simulink model "DAB Converters ude vr"  (R2022a)
settings: Solver=VariableStepAuto  StartTime=0.0  StopTime=0.5  RelTol=1e-3
libraries: spsMosfetLib x16, spsSeriesRLCBranchLib x6, spsVoltageMeasurementLib x6, spsCurrentMeasurementLib x4, simulink_extras x4, spsSawtoothGeneratorLib x4, spspowerguiLib x3, spsControlledVoltageSourceLib x2, spsLinearTransformerLib x2, spsControlledCurrentSourceLib x2, slpidlib x1
settings Model: Creator=shuai  LastModifiedBy=shuai

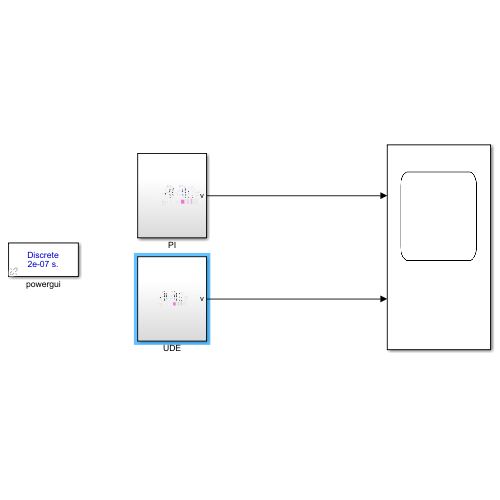
[thumbnail: Simulink's stored preview of the top-level diagram]
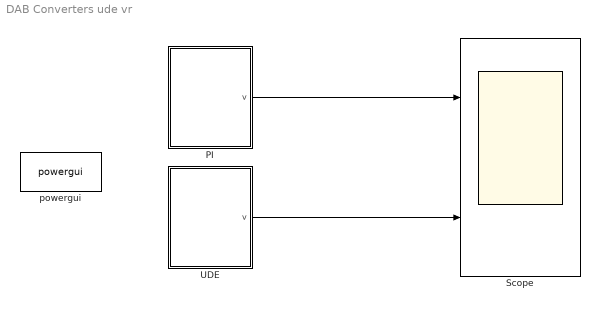
== system DAB Converters ude vr ==
  PI : Subsystem
  Scope : Scope  NumInputPorts=2
  UDE : Subsystem
  powergui : spspowerguiLib/powergui  Priority=1  SimulationMode=Discrete  SampleTime=2e-7  frequency=60  Iterations=50  frequencyindice=0  Pbase=100e6  ErrMax=1e-4  UnitsV=kV  UnitsW=MW  buscounter=0  FunctionMessages=off  echomessages=off  EnableUseOfTLC=off  CurrentSourceSwitches=off  DisableSnubberDevices=off  DisableRonSwitches=off  DisableVfSwitches=off  DisplayEquations=off  AutomaticDiscreteSolvers=off  SolverType=Tustin/Backward Euler (TBE)  Interpol=off  ExternalGateDelay=off  methode=off  Ts=100  x0status=blocks  SPID=on  SwTol=0  HookPort=off  NonlinearTolerance=1e-4  nMaxIteration=100  ContinueOnMaxIteration=off  RestoreLinks=warning  ResistiveCurrentMeasurement=off  Frange=[0:2:500]  Ylog=off  Xlog=on  ShowGrid=off  save=off  variable=ZData  structure=0  ZoomFFT=off  StartTime=0.0  cycles=1  DisplayStyle=1  fundamental=60  FreqAxis=off  MaxFrequency=1000  frequencyindicesteady=1  RmsSteady=1  display=off
  wires:
  PI/1(v) -> Scope/1
  UDE/1(v) -> Scope/2

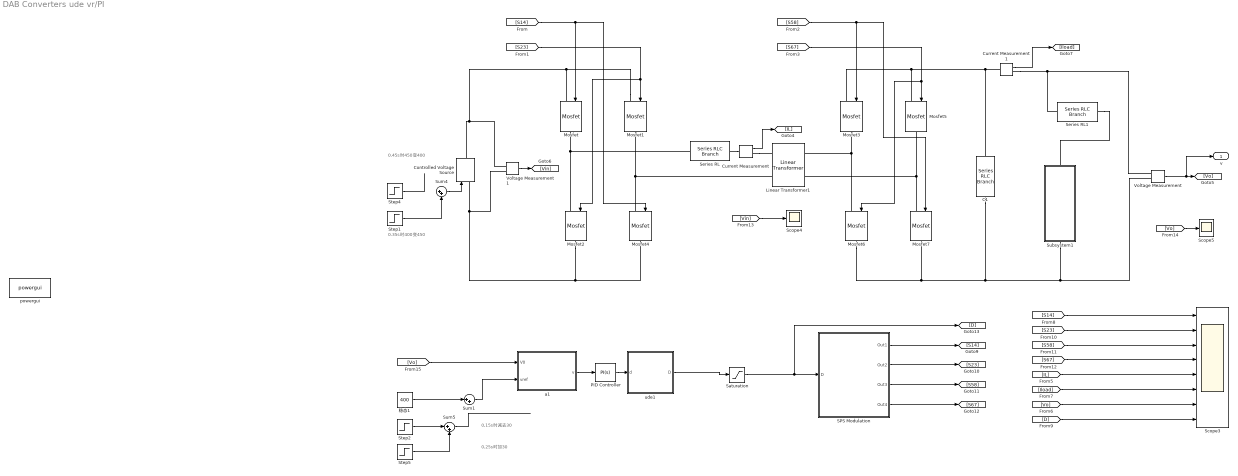
== system DAB Converters ude vr/PI ==
  note: 0.35s时400变450
  note: 0.45s时450变400
  note: 0,25s时加30
  note: 0,15s时减去30
  C1 : spsSeriesRLCBranchLib/Series RLC Branch  LConnTagsString=__new0  RConnTagsString=__new0  BranchType=C  Resistance=0.01  Inductance=1e-3  SetiL0=off  InitialCurrent=0  Capacitance=400e-6  Setx0=on  InitialVoltage=0  Measurements=None
  Controlled Voltage Source : spsControlledVoltageSourceLib/Controlled Voltage Source  Initialize=on  Source_Type=DC  Amplitude=0  Phase=0  Frequency=0  Measurements=None
  Current Measurement : spsCurrentMeasurementLib/Current Measurement  PhasorSimulation=off  OutputType=Complex  PSBequivalent=0
  Current Measurement1 : spsCurrentMeasurementLib/Current Measurement  PhasorSimulation=off  OutputType=Complex  PSBequivalent=0
  Linear Transformer1 : spsLinearTransformerLib/Linear Transformer  UNITS=SI  NominalPower=[20e5 20000 ]  winding1=[1000 0 0]  winding2=[1000 0 0]  ThreeWindings=off  winding3=[3.15e+05 39690 12.634]  RmLm=[8.5e4 8.5e4]  Measurements=None  DataType=on
  Mosfet{,1..7} (8 alike) : spsMosfetLib/Mosfet  Ron=0.001  Lon=0  Rd=0.001  Vfd=0  IC=0  Rs=1e5  Cs=inf  Measurements=off
  PID Controller : slpidlib/PID Controller  Controller=PI  Form=Parallel  TimeDomain=Continuous-time  UseExternalTs=off  SampleTime=-1  IntegratorMethod=Forward Euler  FilterMethod=Forward Euler  ControllerParametersSource=internal  P=0.000544489  I=0.116994  UseKiTs=off  D=0  N=100  UseFilter=on  TunerSelectOption=Transfer Function Based (PID Tuner App)  InitialConditionSource=internal  InitialConditionForIntegrator=0  InitialConditionForFilter=0  DifferentiatorICPrevScaledInput=0  ExternalReset=none  TrackingMode=off  Kt=1  LimitOutput=off  SatLimitsSource=internal  UpperSaturationLimit=inf  LowerSaturationLimit=-inf  LinearizeAsGain=on  AntiWindupMode=none  Kb=1  POutMin=[]  POutMax=[]  IOutMin=[]  IOutMax=[]  DOutMin=[]  DOutMax=[]  NOutMin=[]  NOutMax=[]  SumOutMin=[]  SumOutMax=[]  SaturationOutMin=[]  SaturationOutMax=[]  PParamMin=[]  PParamMax=[]  IParamMin=[]  IParamMax=[]  DParamMin=[]  DParamMax=[]  NParamMin=[]  NParamMax=[]  KbParamMin=[]  KbParamMax=[]  KtParamMin=[]  KtParamMax=[]  KbOutMin=[]  KbOutMax=[]  KtOutMin=[]  KtOutMax=[]  IntegratorOutMin=[]  IntegratorOutMax=[]  FilterOutMin=[]  FilterOutMax=[]  SumI1OutMin=[]  SumI1OutMax=[]  SumI2OutMin=[]  SumI2OutMax=[]  SumI3OutMin=[]  SumI3OutMax=[]  SumI4OutMin=[]  SumI4OutMax=[]  SumDOutMin=[]  SumDOutMax=[]  DifferentiatorOutMin=[]  DifferentiatorOutMax=[]  FilterDiffOutCoefMin=[]  FilterDiffOutCoefMax=[]  ReciprocalOutMin=[]  ReciprocalOutMax=[]  SumDenOutMin=[]  SumDenOutMax=[]  SumNumOutMin=[]  SumNumOutMax=[]  DivideOutMin=[]  DivideOutMax=[]  UdiffTsProdOutMin=[]  UdiffTsProdOutMax=[]  NTsProdOutMin=[]  NTsProdOutMax=[]  UintegralTsProdOutMin=[]  UintegralTsProdOutMax=[]  UngainTsProdOutMin=[]  UngainTsProdOutMax=[]  IntegratorContinuousStateAttributes=''  IntegratorStateMustResolveToSignalObject=off  IntegratorRTWStateStorageClass=Auto  FilterContinuousStateAttributes=''  FilterStateMustResolveToSignalObject=off  FilterRTWStateStorageClass=Auto  ParallelPVariant=InternalParameters  IdealPVariant=Disabled  IVariant=InternalParameters  DVariant=Disabled  IntegratorVariant=Continuous  SatVariant=Disabled  AWVariant=Passthrough  PCopyVariant=Disabled  TRVariant=Disabled  FdbkBlocksVariant=Forward  IdealPFdbkVariant=Disabled  SatFdbkVariant=Disabled  DerivativeFilterVariant=Disabled  NVariant=Disabled  NCopyVariant=Disabled_SignalSpec  FilterICVariant=Disabled  IntegratorICVariant=InternalICs  ExternalResetVariant=Disabled  TRSumVariant=Passthrough  SumFdbkVariant=Disabled  SumVariant=Sum_PI  TsampFilterVariant=InternalTs  TsampNgainVariant=Passthrough  TsampIntegralVariant=Passthrough  ExternalSaturationOutDataTypeStr=Inherit: Same as second input  aMode=0
  SPS Modulation : Subsystem
  Saturation : Saturate  UpperLimit=0.9  LowerLimit=0
  Scope3 : Scope  NumInputPorts=8
  Scope4 : Scope
  Scope5 : Scope
  Series RL : spsSeriesRLCBranchLib/Series RLC Branch  LConnTagsString=__new0  RConnTagsString=__new0  BranchType=L  Resistance=0  Inductance=50e-6  SetiL0=off  InitialCurrent=0  Capacitance=1e-6  Setx0=off  InitialVoltage=0  Measurements=None
  Series RL1 : spsSeriesRLCBranchLib/Series RLC Branch  LConnTagsString=__new0  RConnTagsString=__new0  BranchType=R  Resistance=0.0001  Inductance=50e-6  SetiL0=off  InitialCurrent=0  Capacitance=1e-6  Setx0=off  InitialVoltage=0  Measurements=None
  Step1 : Step  Time=0.3  Before=400  After=400  SampleTime=0
  Step2 : Step  Time=0.1  After=-30  SampleTime=0
  Step4 : Step  Time=0.4  After=-50  SampleTime=0
  Step5 : Step  Time=0.2  After=50  SampleTime=0
  Subsystem1 : Subsystem
  Sum1 : Sum  Inputs=|++
  Sum4 : Sum  Inputs=|++
  Sum5 : Sum  Inputs=|++
  Voltage Measurement : spsVoltageMeasurementLib/Voltage Measurement  PhasorSimulation=off  OutputType=Complex  PSBequivalent=0
  Voltage Measurement1 : spsVoltageMeasurementLib/Voltage Measurement  PhasorSimulation=off  OutputType=Complex  PSBequivalent=0
  a1 : MATLAB Function  TreatAsAtomicUnit=on  SystemSampleTime=1/20000
  powergui : spspowerguiLib/powergui  Priority=1  SimulationMode=Discrete  SampleTime=2e-7  frequency=60  Iterations=50  frequencyindice=0  Pbase=100e6  ErrMax=1e-4  UnitsV=kV  UnitsW=MW  buscounter=0  FunctionMessages=off  echomessages=off  EnableUseOfTLC=off  CurrentSourceSwitches=off  DisableSnubberDevices=off  DisableRonSwitches=off  DisableVfSwitches=off  DisplayEquations=off  AutomaticDiscreteSolvers=off  SolverType=Tustin/Backward Euler (TBE)  Interpol=off  ExternalGateDelay=off  methode=off  Ts=100  x0status=blocks  SPID=off  SwTol=0  HookPort=off  NonlinearTolerance=1e-4  nMaxIteration=100  ContinueOnMaxIteration=off  RestoreLinks=warning  ResistiveCurrentMeasurement=off  Frange=[0:2:500]  Ylog=off  Xlog=on  ShowGrid=off  save=off  variable=ZData  structure=0  ZoomFFT=off  StartTime=0.0  cycles=1  DisplayStyle=1  fundamental=60  FreqAxis=off  MaxFrequency=1000  frequencyindicesteady=1  RmsSteady=1  display=off
  ude1 : MATLAB Function  TreatAsAtomicUnit=on  SystemSampleTime=1/20000
  稳态1 : Constant  Value=400  VectorParams1D=off
  v : Outport
  wires:
  SPS Modulation/4(Out4) -> [S67]
  [S23] -> Scope3/2
  Current Measurement1/1 -> [Iload]
  [S67] -> Mosfet6/1, Mosfet5/1
  SPS Modulation/3(Out3) -> [S58]
  [S58] -> Mosfet7/1, Mosfet3/1
  [S14] -> Scope3/1
  [Vin] -> Scope4/1
  Current Measurement/1 -> [IL]
  Sum4/1 -> Controlled Voltage Source/1
  [D] -> Scope3/8
  Step4/1 -> ?
  Voltage Measurement1/1 -> [Vin]
  [Vo] -> Scope5/1
  Saturation/1 -> [D], SPS Modulation/1(D)
  [S23] -> Mosfet2/1, Mosfet1/1
  Voltage Measurement/1 -> v/1, [Vo]
  SPS Modulation/2(Out2) -> [S23]
  [S14] -> Mosfet4/1, Mosfet/1
  SPS Modulation/1(Out1) -> [S14]
  [S67] -> Scope3/4
  [Iload] -> Scope3/6
  [S58] -> Scope3/3
  Step1/1 -> Sum4/2
  [IL] -> Scope3/5
  [Vo] -> Scope3/7
  Step2/1 -> Sum5/1
  Step5/1 -> Sum5/2
  Sum5/1 -> ?
  稳态1/1 -> Sum1/1
  [Vo] -> a1/1(V0)
  a1/1(v) -> PID Controller/1
  Sum1/1 -> a1/2(vref)
  PID Controller/1 -> ude1/1(d)
  ude1/1(D) -> Saturation/1
  connections:
  Mosfet1/LConn1 -- Voltage Measurement1/LConn1 -- Controlled Voltage Source/RConn1 -- Mosfet/LConn1
  Mosfet4/RConn1 -- Voltage Measurement1/LConn2 -- Controlled Voltage Source/LConn1 -- Mosfet2/RConn1
  Linear Transformer1/RConn2 -- Mosfet7/LConn1 -- Mosfet5/RConn1
  Current Measurement1/LConn1 -- C1/LConn1 -- Mosfet5/LConn1 -- Mosfet3/LConn1
  Current Measurement1/RConn1 -- Series RL1/LConn1 -- Voltage Measurement/LConn1
  Series RL/RConn1 -- Current Measurement/LConn1
  Mosfet2/LConn1 -- Mosfet/RConn1 -- Series RL/LConn1
  Mosfet1/RConn1 -- Mosfet4/LConn1 -- Linear Transformer1/LConn2
  Current Measurement/RConn1 -- Linear Transformer1/LConn1
  Linear Transformer1/RConn1 -- Mosfet6/LConn1 -- Mosfet3/RConn1
  C1/RConn1 -- Mosfet6/RConn1 -- Mosfet7/RConn1 -- Subsystem1/RConn1 -- Voltage Measurement/LConn2
  Series RL1/RConn1 -- Subsystem1/LConn1

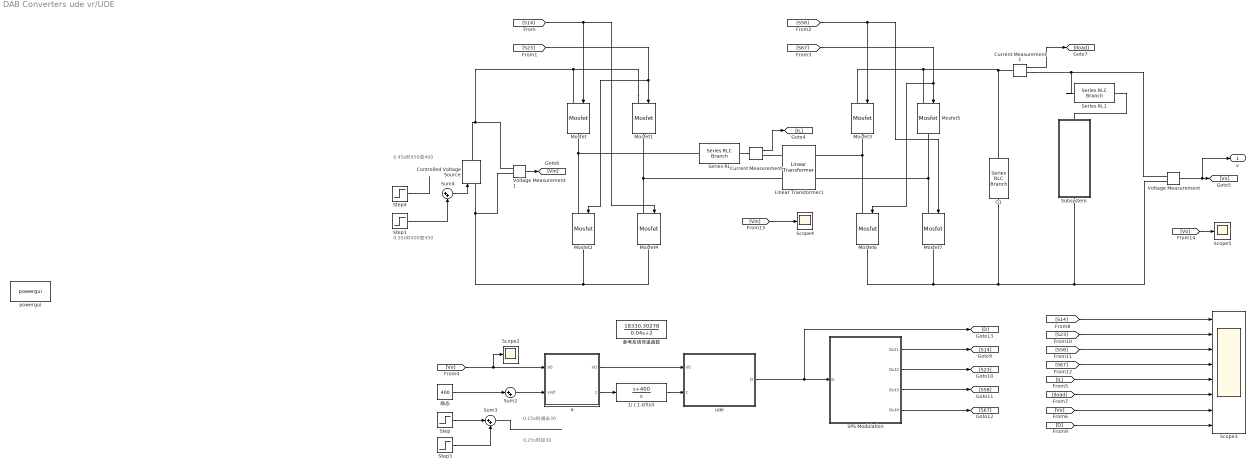
== system DAB Converters ude vr/UDE ==
  note: 0.35s时400变450
  note: 0,15s时减去30
  note: 0,25s时加30
  note: 0.45s时450变400
  1/（1-Gf(s)) : TransferFcn  Numerator=[1 400]  Denominator=[1 0]
  C1 : spsSeriesRLCBranchLib/Series RLC Branch  LConnTagsString=__new0  RConnTagsString=__new0  BranchType=C  Resistance=0.01  Inductance=1e-3  SetiL0=off  InitialCurrent=0  Capacitance=400e-6  Setx0=on  InitialVoltage=0  Measurements=None
  Controlled Voltage Source : spsControlledVoltageSourceLib/Controlled Voltage Source  Initialize=on  Source_Type=DC  Amplitude=0  Phase=0  Frequency=0  Measurements=None
  Current Measurement : spsCurrentMeasurementLib/Current Measurement  PhasorSimulation=off  OutputType=Complex  PSBequivalent=0
  Current Measurement1 : spsCurrentMeasurementLib/Current Measurement  PhasorSimulation=off  OutputType=Complex  PSBequivalent=0
  Linear Transformer1 : spsLinearTransformerLib/Linear Transformer  UNITS=SI  NominalPower=[20e5 20000 ]  winding1=[1000 0 0]  winding2=[1000 0 0]  ThreeWindings=off  winding3=[3.15e+05 39690 12.634]  RmLm=[8.5e4 8.5e4]  Measurements=None  DataType=on
  Mosfet{,1..7} (8 alike) : spsMosfetLib/Mosfet  Ron=0.001  Lon=0  Rd=0.001  Vfd=0  IC=0  Rs=1e5  Cs=inf  Measurements=off
  SPS Modulation : Subsystem
  Scope2 : Scope
  Scope3 : Scope  NumInputPorts=8
  Scope4 : Scope
  Scope5 : Scope
  Series RL : spsSeriesRLCBranchLib/Series RLC Branch  LConnTagsString=__new0  RConnTagsString=__new0  BranchType=L  Resistance=0  Inductance=50e-6  SetiL0=off  InitialCurrent=0  Capacitance=1e-6  Setx0=off  InitialVoltage=0  Measurements=None
  Series RL1 : spsSeriesRLCBranchLib/Series RLC Branch  LConnTagsString=__new0  RConnTagsString=__new0  BranchType=R  Resistance=0.0001  Inductance=50e-6  SetiL0=off  InitialCurrent=0  Capacitance=1e-6  Setx0=off  InitialVoltage=0  Measurements=None
  Step : Step  Time=0.1  After=-30  SampleTime=0
  Step1 : Step  Time=0.3  Before=400  After=400  SampleTime=0
  Step3 : Step  Time=0.2  After=50  SampleTime=0
  Step4 : Step  Time=0.4  After=-50  SampleTime=0
  Subsystem : Subsystem
  Sum2 : Sum  Inputs=|++
  Sum3 : Sum  Inputs=|++
  Sum4 : Sum  Inputs=|++
  Voltage Measurement : spsVoltageMeasurementLib/Voltage Measurement  PhasorSimulation=off  OutputType=Complex  PSBequivalent=0
  Voltage Measurement1 : spsVoltageMeasurementLib/Voltage Measurement  PhasorSimulation=off  OutputType=Complex  PSBequivalent=0
  a : MATLAB Function  TreatAsAtomicUnit=on  SystemSampleTime=1/20000
  powergui : spspowerguiLib/powergui  Priority=1  SimulationMode=Discrete  SampleTime=2e-7  frequency=60  Iterations=50  frequencyindice=0  Pbase=100e6  ErrMax=1e-4  UnitsV=kV  UnitsW=MW  buscounter=0  FunctionMessages=off  echomessages=off  EnableUseOfTLC=off  CurrentSourceSwitches=off  DisableSnubberDevices=off  DisableRonSwitches=off  DisableVfSwitches=off  DisplayEquations=off  AutomaticDiscreteSolvers=off  SolverType=Tustin/Backward Euler (TBE)  Interpol=off  ExternalGateDelay=off  methode=off  Ts=100  x0status=blocks  SPID=off  SwTol=0  HookPort=off  NonlinearTolerance=1e-4  nMaxIteration=100  ContinueOnMaxIteration=off  RestoreLinks=warning  ResistiveCurrentMeasurement=off  Frange=[0:2:500]  Ylog=off  Xlog=on  ShowGrid=off  save=off  variable=ZData  structure=0  ZoomFFT=off  StartTime=0.0  cycles=1  DisplayStyle=1  fundamental=60  FreqAxis=off  MaxFrequency=1000  frequencyindicesteady=1  RmsSteady=1  display=off
  ude : MATLAB Function  TreatAsAtomicUnit=on  SystemSampleTime=1/20000
  参考系统传递函数 : TransferFcn  Numerator=[18330.30278]  Denominator=[0.04 2]
  稳态 : Constant  Value=400  VectorParams1D=off
  v : Outport
  wires:
  SPS Modulation/4(Out4) -> [S67]
  [S23] -> Scope3/2
  Current Measurement1/1 -> [Iload]
  [S67] -> Mosfet6/1, Mosfet5/1
  SPS Modulation/3(Out3) -> [S58]
  [S58] -> Mosfet7/1, Mosfet3/1
  [S14] -> Scope3/1
  [Vin] -> Scope4/1
  Current Measurement/1 -> [IL]
  Sum4/1 -> Controlled Voltage Source/1
  [D] -> Scope3/8
  1/（1-Gf(s))/1 -> ude/2(z)
  稳态/1 -> Sum2/1
  Sum2/1 -> a/2(vref)
  Step4/1 -> ?
  Voltage Measurement1/1 -> [Vin]
  [Vo] -> Scope5/1
  ude/1(D) -> [D], SPS Modulation/1(D)
  [S23] -> Mosfet2/1, Mosfet1/1
  a/1(V0) -> ude/1(V0)
  Step/1 -> Sum3/1
  Voltage Measurement/1 -> v/1, [Vo]
  a/2(z) -> 1/（1-Gf(s))/1
  SPS Modulation/2(Out2) -> [S23]
  [S14] -> Mosfet4/1, Mosfet/1
  SPS Modulation/1(Out1) -> [S14]
  [S67] -> Scope3/4
  [Iload] -> Scope3/6
  [S58] -> Scope3/3
  Step1/1 -> Sum4/2
  [Vo] -> a/1("V0 "), Scope2/1
  Sum3/1 -> ?
  Step3/1 -> Sum3/2
  [IL] -> Scope3/5
  [Vo] -> Scope3/7
  connections:
  Mosfet1/LConn1 -- Voltage Measurement1/LConn1 -- Controlled Voltage Source/RConn1 -- Mosfet/LConn1
  Mosfet4/RConn1 -- Voltage Measurement1/LConn2 -- Controlled Voltage Source/LConn1 -- Mosfet2/RConn1
  Linear Transformer1/RConn2 -- Mosfet7/LConn1 -- Mosfet5/RConn1
  Current Measurement1/LConn1 -- C1/LConn1 -- Mosfet5/LConn1 -- Mosfet3/LConn1
  Series RL/RConn1 -- Current Measurement/LConn1
  Mosfet2/LConn1 -- Series RL/LConn1 -- Mosfet/RConn1
  Mosfet1/RConn1 -- Mosfet4/LConn1 -- Linear Transformer1/LConn2
  Current Measurement/RConn1 -- Linear Transformer1/LConn1
  Linear Transformer1/RConn1 -- Mosfet6/LConn1 -- Mosfet3/RConn1
  C1/RConn1 -- Mosfet6/RConn1 -- Mosfet7/RConn1 -- Voltage Measurement/LConn2 -- Subsystem/RConn1
  Current Measurement1/RConn1 -- Series RL1/LConn1 -- Voltage Measurement/LConn1
  Series RL1/RConn1 -- Subsystem/LConn1

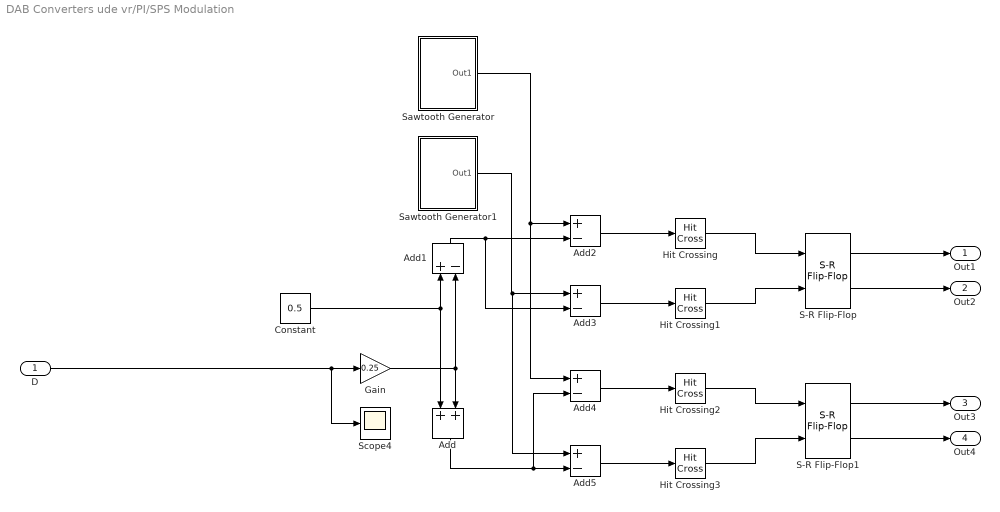
== system DAB Converters ude vr/PI/SPS Modulation ==
  D : Inport
  Add : Sum
  Add{1..5} (5 alike) : Sum  Inputs=+-
  Constant : Constant  Value=0.5
  Gain : Gain  Gain=0.25
  Hit Crossing{,1..3} (4 alike) : HitCross  HitCrossingDirection=rising
  S-R Flip-Flop : simulink_extras/Flip Flops/S-R Flip-Flop  initial_condition=0
  S-R Flip-Flop1 : simulink_extras/Flip Flops/S-R Flip-Flop  initial_condition=0
  Sawtooth Generator : Subsystem  mask{fs=20000}
      mask prompts: fs "Frequency (Hz)"
      mask help: Sawtooth Generator
  Sawtooth Generator1 : Subsystem  mask{fs=20000}
      mask prompts: fs "Frequency (Hz)"
      mask help: Sawtooth Generator
  Scope4 : Scope
  Out1 : Outport  VectorParamsAs1DForOutWhenUnconnected=off
  Out2 : Outport  Port=2  VectorParamsAs1DForOutWhenUnconnected=off
  Out3 : Outport  Port=3  VectorParamsAs1DForOutWhenUnconnected=off
  Out4 : Outport  Port=4  VectorParamsAs1DForOutWhenUnconnected=off
  wires:
  Hit Crossing1/1 -> S-R Flip-Flop/2
  Add1/1 -> Add3/2, Add2/2
  Constant/1 -> Add1/1, Add/1
  Add5/1 -> Hit Crossing3/1
  Gain/1 -> Add1/2, Add/2
  D/1 -> Gain/1, Scope4/1
  Add/1 -> Add4/2, Add5/2
  Sawtooth Generator/1(Out1) -> Add4/1, Add2/1
  Hit Crossing/1 -> S-R Flip-Flop/1
  Add2/1 -> Hit Crossing/1
  Sawtooth Generator1/1(Out1) -> Add5/1, Add3/1
  Add3/1 -> Hit Crossing1/1
  Add4/1 -> Hit Crossing2/1
  Hit Crossing2/1 -> S-R Flip-Flop1/1
  Hit Crossing3/1 -> S-R Flip-Flop1/2
  S-R Flip-Flop1/1 -> Out3/1
  S-R Flip-Flop1/2 -> Out4/1
  S-R Flip-Flop/1 -> Out1/1
  S-R Flip-Flop/2 -> Out2/1

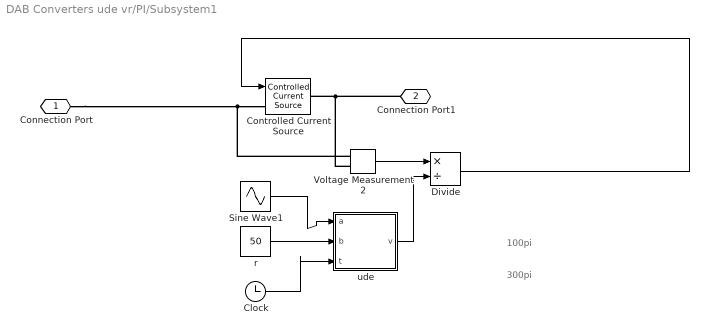
== system DAB Converters ude vr/PI/Subsystem1 ==
  note: 300pi
  note: 100pi
  Clock : Clock
  Controlled Current Source : spsControlledCurrentSourceLib/Controlled Current Source  Initialize=on  Source_Type=AC  Amplitude=0  Phase=0  Frequency=0  Measurements=None
  Divide : Product  Inputs=*/  RndMeth=Zero  SaturateOnIntegerOverflow=on
  Sine Wave1 : Sin  Amplitude=10  Bias=50  Frequency=100*pi  Samples=1e5  SampleTime=0
  Voltage Measurement2 : spsVoltageMeasurementLib/Voltage Measurement  PhasorSimulation=off  OutputType=Complex  PSBequivalent=0
  r : Constant  Value=50  VectorParams1D=off
  ude : MATLAB Function  TreatAsAtomicUnit=on  SystemSampleTime=1/20000
  Connection Port : PMIOPort  Side=Left
  Connection Port1 : PMIOPort  Port=2  Side=Right
  wires:
  Voltage Measurement2/1 -> Divide/1
  Sine Wave1/1 -> ude/1(a)
  Divide/1 -> Controlled Current Source/1
  Clock/1 -> ude/3(t)
  r/1 -> ude/2(b)
  ude/1(v) -> Divide/2
  connections:
  Voltage Measurement2/LConn2 -- Connection Port1/RConn1 -- Controlled Current Source/RConn1
  Voltage Measurement2/LConn1 -- Connection Port/RConn1 -- Controlled Current Source/LConn1

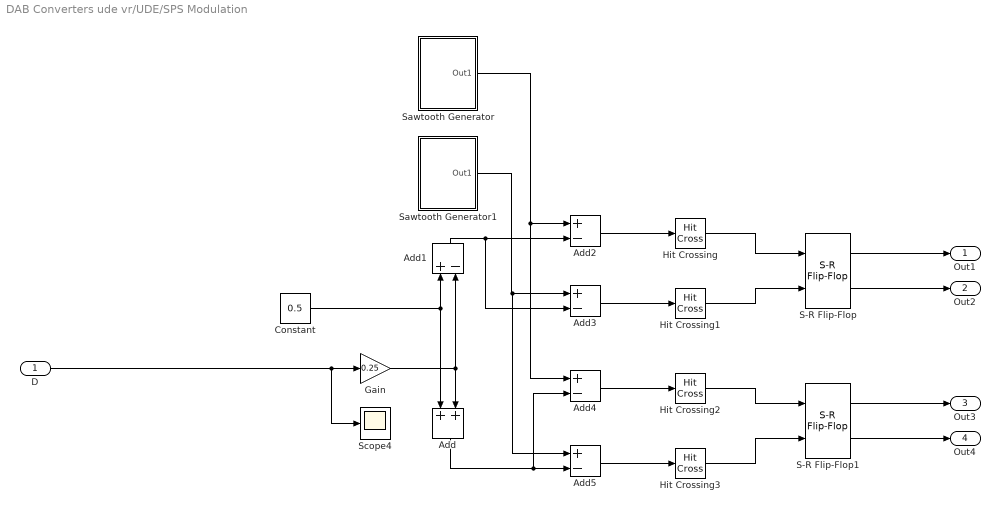
== system DAB Converters ude vr/UDE/SPS Modulation ==
  D : Inport
  Add : Sum
  Add{1..5} (5 alike) : Sum  Inputs=+-
  Constant : Constant  Value=0.5
  Gain : Gain  Gain=0.25
  Hit Crossing{,1..3} (4 alike) : HitCross  HitCrossingDirection=rising
  S-R Flip-Flop : simulink_extras/Flip Flops/S-R Flip-Flop  initial_condition=0
  S-R Flip-Flop1 : simulink_extras/Flip Flops/S-R Flip-Flop  initial_condition=0
  Sawtooth Generator : Subsystem  mask{fs=20000}
      mask prompts: fs "Frequency (Hz)"
      mask help: Sawtooth Generator
  Sawtooth Generator1 : Subsystem  mask{fs=20000}
      mask prompts: fs "Frequency (Hz)"
      mask help: Sawtooth Generator
  Scope4 : Scope
  Out1 : Outport  VectorParamsAs1DForOutWhenUnconnected=off
  Out2 : Outport  Port=2  VectorParamsAs1DForOutWhenUnconnected=off
  Out3 : Outport  Port=3  VectorParamsAs1DForOutWhenUnconnected=off
  Out4 : Outport  Port=4  VectorParamsAs1DForOutWhenUnconnected=off
  wires:
  Hit Crossing1/1 -> S-R Flip-Flop/2
  Add1/1 -> Add3/2, Add2/2
  Constant/1 -> Add1/1, Add/1
  Add5/1 -> Hit Crossing3/1
  Gain/1 -> Add1/2, Add/2
  D/1 -> Gain/1, Scope4/1
  Add/1 -> Add4/2, Add5/2
  Sawtooth Generator/1(Out1) -> Add4/1, Add2/1
  Hit Crossing/1 -> S-R Flip-Flop/1
  Add2/1 -> Hit Crossing/1
  Sawtooth Generator1/1(Out1) -> Add5/1, Add3/1
  Add3/1 -> Hit Crossing1/1
  Add4/1 -> Hit Crossing2/1
  Hit Crossing2/1 -> S-R Flip-Flop1/1
  Hit Crossing3/1 -> S-R Flip-Flop1/2
  S-R Flip-Flop1/1 -> Out3/1
  S-R Flip-Flop1/2 -> Out4/1
  S-R Flip-Flop/1 -> Out1/1
  S-R Flip-Flop/2 -> Out2/1

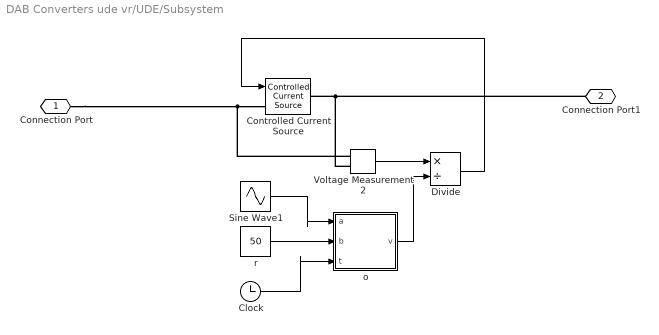
== system DAB Converters ude vr/UDE/Subsystem ==
  Clock : Clock
  Controlled Current Source : spsControlledCurrentSourceLib/Controlled Current Source  Initialize=on  Source_Type=AC  Amplitude=0  Phase=0  Frequency=0  Measurements=None
  Divide : Product  Inputs=*/  RndMeth=Zero  SaturateOnIntegerOverflow=on
  Sine Wave1 : Sin  Amplitude=10  Bias=50  Frequency=100*pi  Samples=1e5  SampleTime=0
  Voltage Measurement2 : spsVoltageMeasurementLib/Voltage Measurement  PhasorSimulation=off  OutputType=Complex  PSBequivalent=0
  o : MATLAB Function  TreatAsAtomicUnit=on  SystemSampleTime=1/20000
  r : Constant  Value=50  VectorParams1D=off
  Connection Port : PMIOPort  Side=Left
  Connection Port1 : PMIOPort  Port=2  Side=Right
  wires:
  Voltage Measurement2/1 -> Divide/1
  Sine Wave1/1 -> o/1(a)
  Divide/1 -> Controlled Current Source/1
  Clock/1 -> o/3(t)
  r/1 -> o/2(b)
  o/1(v) -> Divide/2
  connections:
  Voltage Measurement2/LConn2 -- Connection Port1/RConn1 -- Controlled Current Source/RConn1
  Voltage Measurement2/LConn1 -- Connection Port/RConn1 -- Controlled Current Source/LConn1

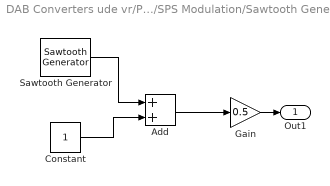
== system DAB Converters ude vr/PI/SPS Modulation/Sawtooth Generator ==
  Add : Sum
  Constant : Constant
  Gain : Gain  Gain=0.5
  Sawtooth Generator : spsSawtoothGeneratorLib/Sawtooth Generator  Freq=fs  Phase=180  Ts=0
  Out1 : Outport  VectorParamsAs1DForOutWhenUnconnected=off
  wires:
  Add/1 -> Gain/1
  Gain/1 -> Out1/1
  Constant/1 -> Add/2
  Sawtooth Generator/1 -> Add/1

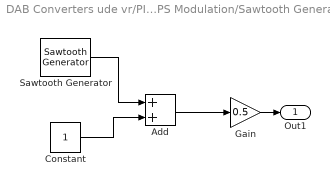
== system DAB Converters ude vr/PI/SPS Modulation/Sawtooth Generator1 ==
  Add : Sum
  Constant : Constant
  Gain : Gain  Gain=0.5
  Sawtooth Generator : spsSawtoothGeneratorLib/Sawtooth Generator  Freq=fs  Phase=0  Ts=0
  Out1 : Outport  VectorParamsAs1DForOutWhenUnconnected=off
  wires:
  Add/1 -> Gain/1
  Gain/1 -> Out1/1
  Constant/1 -> Add/2
  Sawtooth Generator/1 -> Add/1

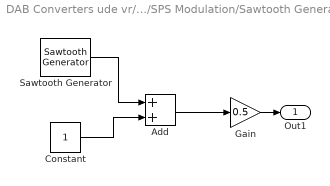
== system DAB Converters ude vr/UDE/SPS Modulation/Sawtooth Generator ==
  Add : Sum
  Constant : Constant
  Gain : Gain  Gain=0.5
  Sawtooth Generator : spsSawtoothGeneratorLib/Sawtooth Generator  Freq=fs  Phase=180  Ts=0
  Out1 : Outport  VectorParamsAs1DForOutWhenUnconnected=off
  wires:
  Add/1 -> Gain/1
  Gain/1 -> Out1/1
  Constant/1 -> Add/2
  Sawtooth Generator/1 -> Add/1

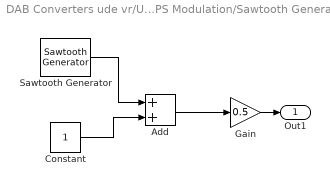
== system DAB Converters ude vr/UDE/SPS Modulation/Sawtooth Generator1 ==
  Add : Sum
  Constant : Constant
  Gain : Gain  Gain=0.5
  Sawtooth Generator : spsSawtoothGeneratorLib/Sawtooth Generator  Freq=fs  Phase=0  Ts=0
  Out1 : Outport  VectorParamsAs1DForOutWhenUnconnected=off
  wires:
  Add/1 -> Gain/1
  Gain/1 -> Out1/1
  Constant/1 -> Add/2
  Sawtooth Generator/1 -> Add/1

== matlab function DAB Converters ude vr/UDE/Subsystem/o ==
  data: a input; v output; b input; t input
function v = fcn(a,b,t)

if(t>0.1)
    v=a;
else 
    v=b;
end

== matlab function DAB Converters ude vr/PI/Subsystem1/ude ==
  data: a input; v output; b input; t input
function v = fcn(a,b,t)

if(t>0.1)
    v=a;
else 
    v=b;
end

== matlab function DAB Converters ude vr/UDE/a ==
  data: V0 output; V0 input; z output; vref input
function [V0,z] = fcn(V0,vref)

Am=-400;%%Xm点=-αXm(t)+-αC(t)
Bm=400;%%
k=0;
vowen=400;
v=V0-vowen;
c=vref-vowen;%%c为相较于稳态时期望电压的变化值
e=c-v;
z=Am*v+Bm*c-k*e;

== matlab function DAB Converters ude vr/UDE/ude ==
  data: V0 input; D output; z input
function D = fcn(V0,z)
fs=20e3;%%工作频率
n=1;
C=400e-6;%%输出端电容
L=50e-6;%%电感
V1=400;%%输入电压
R=50;%%输出端电压
D1=0.5-0.1*sqrt(21);%%当输出电压为400v时，根据输处电压与输入d之间的关系求得
A=-1/(R*C);
B=n*(1-2*D1)*V1/(2*fs*L*C);%%小信号建模后，D1为稳态值时输出电压
vowen=400;
beita=400;%%   Gf（s）= β/(s+β) 中的β
v=V0-vowen;%% v为电压相对于第一次稳态时的变压变化，vowen为第一次稳态的电压，Vo为输出电压
d=(-1/B)*(A*v+v*beita-z);%%z
D=D1+d;

== matlab function DAB Converters ude vr/PI/a1 ==
  data: V0 input; v output; vref input
function v = fcn(V0,vref)

vowen=400;
ve=V0-vowen;
c=vref-vowen;%%c为相较于稳态时期望电压的变化值
v=c-ve;

== matlab function DAB Converters ude vr/PI/ude1 ==
  data: d input; D output
function D = fcn(d)
D1=0.5-0.1*sqrt(21);
D=D1+d;
